simulink model "Demo_2"  (R2024b)
settings: Solver=FixedStepAuto  StartTime=0.0  StopTime=20.0  FixedStep=0.01  RelTol=1e-3
libraries: simulink x2, SignalEditorBlockLib x1
settings Model: Creator=Marcin  LastModifiedBy=Marcin

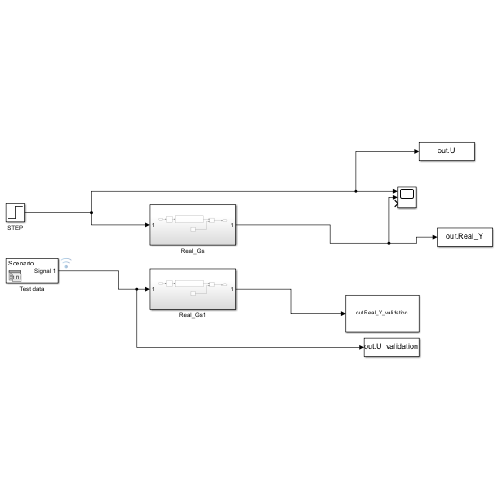
[thumbnail: Simulink's stored preview of the top-level diagram]
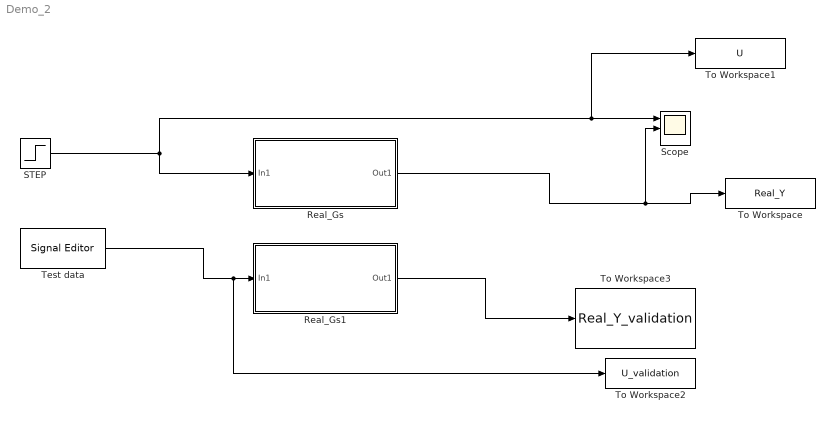
== system Demo_2 ==
  Real_Gs : Subsystem
  Real_Gs1 : Subsystem
  STEP : Step  SampleTime=0
  Scope : Scope  NumInputPorts=3
  Test data : SignalEditorBlockLib/Signal Editor  FileName=test_excitation_signal.mat  ActiveScenario=Scenario  ActiveSignal=Signal 1  IsBus=off  OutputBusObjectStr=Bus: BusObject  SampleTime=0  Interpolate=off  ZeroCross=off  OutputAfterFinalValue=Setting to zero  Unit=inherit  PreserveSignalName=on  ApplySigPropsToAllScenarios=on  ApplySigPropsToAllSignals=off
  To Workspace : ToWorkspace  VariableName=Real_Y  SaveFormat=Timeseries  SampleTime=-1
  To Workspace1 : ToWorkspace  VariableName=U  SaveFormat=Timeseries  SampleTime=-1
  To Workspace2 : ToWorkspace  VariableName=U_validation  SaveFormat=Timeseries  SampleTime=-1
  To Workspace3 : ToWorkspace  VariableName=Real_Y_validation  SaveFormat=Timeseries  SampleTime=-1
  wires:
  STEP/1 -> Real_Gs/1(In1), To Workspace1/1, Scope/1
  Real_Gs/1(Out1) -> Scope/2, To Workspace/1
  Test data/1 -> To Workspace2/1, Real_Gs1/1(In1)
  Real_Gs1/1(Out1) -> To Workspace3/1

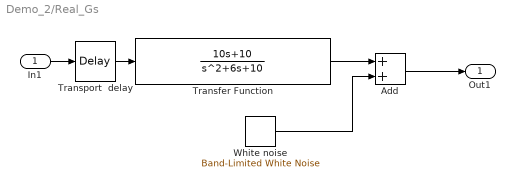
== system Demo_2/Real_Gs ==
  In1 : Inport
  Add : Sum
  Transfer Function : TransferFcn  Numerator=[10 10]  Denominator=[1 6 10]
  Transport  delay : TransportDelay  DelayTime=2
  White noise : simulink/Sources/Band-Limited White Noise  Cov=[0.00001]  Ts=0.01  seed=[23323441]
  Out1 : Outport
  wires:
  Transport  delay/1 -> Transfer Function/1
  Transfer Function/1 -> Add/1
  White noise/1 -> Add/2
  In1/1 -> Transport  delay/1
  Add/1 -> Out1/1

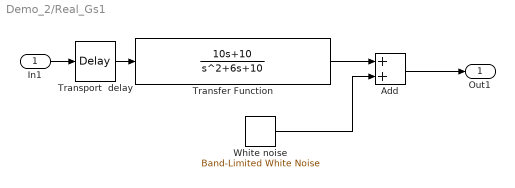
== system Demo_2/Real_Gs1 ==
  In1 : Inport
  Add : Sum
  Transfer Function : TransferFcn  Numerator=[10 10]  Denominator=[1 6 10]
  Transport  delay : TransportDelay  DelayTime=2
  White noise : simulink/Sources/Band-Limited White Noise  Cov=[0.00001]  Ts=0.01  seed=[23323441]
  Out1 : Outport
  wires:
  Transport  delay/1 -> Transfer Function/1
  Transfer Function/1 -> Add/1
  White noise/1 -> Add/2
  In1/1 -> Transport  delay/1
  Add/1 -> Out1/1
